simulink model "adm1_ss"  (R2021b)
settings: Solver=ode15s  StartTime=0.0  StopTime=600  FixedStep=0.01  RelTol=1e-5  AbsTol=1e-8
settings Model: Creator=ielulf  LastModifiedBy=javanmcguckin
settings SolverCC: AutoScaleAbsTol=off  AlgebraicLoopSolver=TrustRegion
settings DataIOCC: InitialState=xFinal  SaveFormat=Array  SignalLoggingSaveFormat=ModelDataLogs  SaveOutput=off  ReturnWorkspaceOutputs=off  TimeSaveName=t  SignalLoggingName=sigsOut  OutputTimes=[0:(1/96):609]
settings OptimizationCC: BlockReduction=off  BooleanDataType=off  OptimizeBlockIOStorage=off  BufferReuse=off  GlobalBufferReuse=off  ExpressionFolding=off  ExpressionDepthLimit=2147483647  LocalBlockOutputs=off  InitFltsAndDblsToZero=on  LifeSpan=inf
settings DebuggingCC: SaveWithParameterizedLinksMsg=none  UnderspecifiedInitializationDetection=Classic  MergeDetectMultiDrivingBlocksExec=none  SignalResolutionControl=TryResolveAllWithWarning  InheritedTsInSrcMsg=none  MultiTaskDSMMsg=warning  MultiTaskCondExecSysMsg=none  FcnCallInpInsideContextMsg=warning  UnconnectedOutputMsg=none  StateNameClashWarn=warning  SFUnexpectedBacktrackingDiag=warning  SFNoUnconditionalDefaultTransitionDiag=warning  SFExecutionAtInitializationDiag=none  SFMachineParentedDataDiag=warning  ArithmeticOperatorsInVariantConditions=warning
settings HardwareCC: ProdBitPerPointer=32  ProdBitPerSizeT=32  ProdBitPerPtrDiffT=32  ProdLargestAtomicFloat=None  ProdIntDivRoundTo=Undefined  ProdEndianess=Unspecified  ProdWordSize=32  ProdHWDeviceType=32-bit Generic  TargetUnknown=on
settings ModelReferenceCC: PropagateSignalLabelsOutOfModel=off
settings SFSimCC: SimUseLocalCustomCode=off  CustomCodeUndefinedFunction=UseInterfaceOnly
settings RTWCC: TemplateMakefile=grt_unix.tmf  RTWUseLocalCustomCode=off
settings CodeAppCC: StateflowObjectComments=on
settings GRTTargetCC: TargetFcnLib=ansi_tfl_tmw.mat  TargetLangStandard=C89/C90 (ANSI)  CombineOutputUpdateFcns=off  GRTInterface=on
settings ConfigComp: CovMetricSettings=dw  CovSaveCumulativeToWorkspaceVar=on  CovSaveSingleToWorkspaceVar=on  CovExternalEMLEnable=off

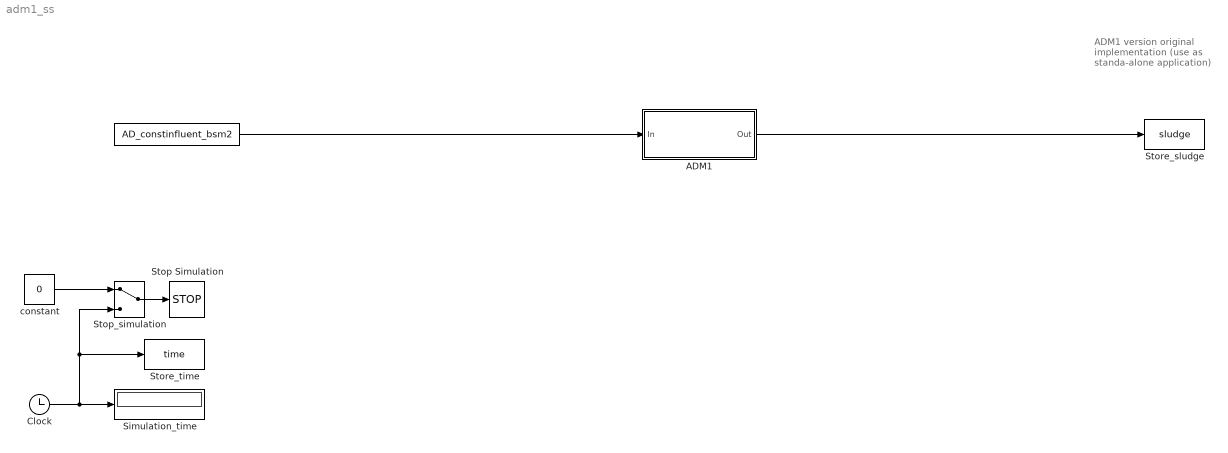
== system adm1_ss ==
  note: ADM1 version
      | original implementation
      | (use as standa-alone application)
  " " : FromWorkspace  VariableName=AD_constinfluent_bsm2  SampleTime=-1  ZeroCross=off  OutputAfterFinalValue=Holding final value
  " constant" : Constant  Value=0
  ADM1 : Subsystem
      mask Display: disp('adm1_ODE_bsm2')
  Clock : Clock
  Simulation_time : Display
  Stop Simulation : Stop
  Stop_simulation : ManualSwitch
  Store_sludge : ToWorkspace  VariableName=sludge
  Store_time : ToWorkspace  VariableName=time
  wires:
  Clock/1 -> Simulation_time/1, Stop_simulation/2, Store_time/1
  Stop_simulation/1 -> Stop Simulation/1
  " constant"/1 -> Stop_simulation/1
  " "/1 -> ADM1/1(In)
  ADM1/1(Out) -> Store_sludge/1

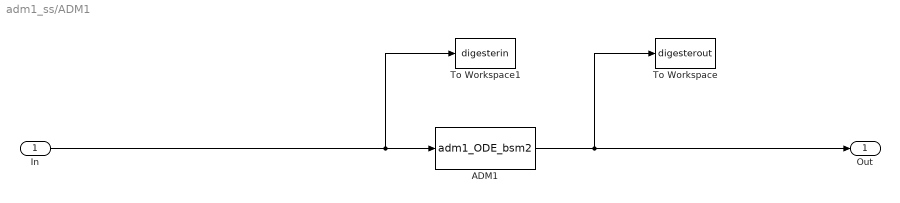
== system adm1_ss/ADM1 ==
  In : Inport
  ADM1 : S-Function  FunctionName=adm1_ODE_bsm2  Parameters=DIGESTERINIT, DIGESTERPAR, DIM_D  SFunctionDeploymentMode=off  EnableBusSupport=off
  To Workspace : ToWorkspace  VariableName=digesterout
  To Workspace1 : ToWorkspace  VariableName=digesterin
  Out : Outport
  wires:
  In/1 -> ADM1/1, To Workspace1/1
  ADM1/1 -> Out/1, To Workspace/1
